simulink model "DesDyn"  (R2023b)
settings: Solver=VariableStepAuto  StartTime=0.0  StopTime=8  RelTol=1e-3
values from neighbouring files (symbols this model uses):
  K_rate = 4*ones(4,1)    [plot_K_pqr.m]    (also in runsim_K_pqr.m = 8*ones(4,1); runsim_K_q.m = 8*ones(4,1))
  tdoublet = 2.5    [plot_K_pqr.m]    (also in runsim_K_pqr.m = 3)
  tstep = 0.1    [plot_K_pqr.m]    (also in runsim_K_pqr.m)
settings Model: Creator=suvo  LastModifiedBy=suvo
settings DataIOCC: ReturnWorkspaceOutputs=off

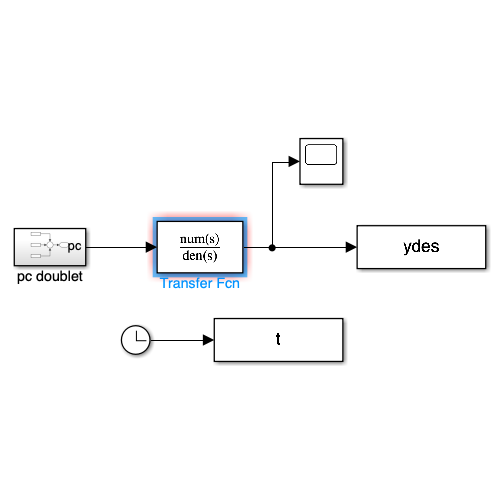
[thumbnail: Simulink's stored preview of the top-level diagram]
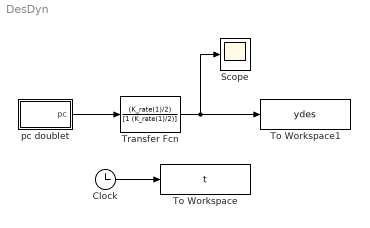
== system DesDyn ==
  Clock : Clock
  Scope : Scope
  To Workspace : ToWorkspace  VariableName=t  SampleTime=-1
  To Workspace1 : ToWorkspace  VariableName=ydes  SampleTime=-1
  Transfer Fcn : TransferFcn  Numerator=(K_rate(1)/2)  Denominator=[1 (K_rate(1)/2)]
  pc doublet : Subsystem
  wires:
  pc doublet/1(pc) -> Transfer Fcn/1
  Transfer Fcn/1 -> To Workspace1/1, Scope/1
  Clock/1 -> To Workspace/1

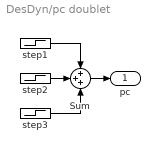
== system DesDyn/pc doublet ==
  Sum : Sum  Inputs=+++
  step1 : Step  Time=tstep  After=10  SampleTime=0
  step2 : Step  Time=tstep+tdoublet  After=-20  SampleTime=0
  step3 : Step  Time=tstep+2*tdoublet  After=10  SampleTime=0
  pc : Outport
  wires:
  Sum/1 -> pc/1
  step1/1 -> Sum/1
  step2/1 -> Sum/2
  step3/1 -> Sum/3
